simulink model "gm_gm_Encoder_test_interface"  (R2021b)
settings: Solver=FixedStepAuto  StartTime=0.0  StopTime=inf  RelTol=1e-3  EnableMultiTasking=on
undefined symbols (not defined in the file or in its folder): AXI4, Lite
libraries: axiinterfacelib x5, simulink x2
settings Model: Creator=Stijn  LastModifiedBy=Jeedella
settings SolverCC: ConcurrentTasks=on  AlgebraicLoopSolver=TrustRegion  PositivePriorityOrder=on
settings DataIOCC: ReturnWorkspaceOutputs=off
settings OptimizationCC: BlockReduction=off  ConditionallyExecuteInputs=off  EnhancedBackFolding=on  PassReuseOutputArgsAs=Individual arguments  MaxStackSize=64  OptimizeBlockOrder=speed  DifferentSizesBufferReuse=on  OptimizationCustomize=off  EfficientTunableParamExpr=on
settings DebuggingCC: AlgebraicLoopMsg=error  InheritedTsInSrcMsg=none  ParameterTunabilityLossMsg=error  SFMachineParentedDataDiag=warning  ArithmeticOperatorsInVariantConditions=warning
settings HardwareCC: ProdBitPerPointer=32  ProdBitPerSizeT=32  ProdBitPerPtrDiffT=32  ProdLargestAtomicInteger=Long  ProdLargestAtomicFloat=Double  ProdWordSize=32  ProdLongLongMode=on  ProdHWDeviceType=ARM Compatible->ARM Cortex  TargetBitPerPointer=64  TargetBitPerSizeT=64  TargetBitPerPtrDiffT=64  TargetLongLongMode=on  TargetIntDivRoundTo=Zero  TargetEndianess=LittleEndian  TargetWordSize=64  TargetHWDeviceType=Custom Processor->MATLAB Host Computer
settings ModelReferenceCC: ModelReferenceNumInstancesAllowed=Single
settings SFSimCC: MATLABDynamicMemAlloc=off  CustomCodeUndefinedFunction=UseInterfaceOnly
settings RTWCC: Description=Embedded Coder  SystemTargetFile=ert.tlc  HardwareBoard=Xilinx Zynq-7000 based board  TLCOptions="-aInlineSetEventsForThisBaseRateFcn=TLC_FALSE -aSuppressMultiTaskScheduler=TLC_FALSE  -aRateBasedStepFcn=0"  TemplateMakefile=ert_default_tmf  GenerateReport=on  Toolchain=Linaro AArch32 Linux v6.3.1  IncludeHyperlinkInReport=on  LaunchReport=on  GenerateTraceInfo=on  GenerateTraceReport=on  GenerateTraceReportSl=on  GenerateTraceReportSf=on  GenerateTraceReportEml=on
settings CodeAppCC: ForceParamTrailComments=on  IgnoreCustomStorageClasses=off  OperatorAnnotations=on  SimulinkDataObjDesc=on  SFDataObjDesc=on  InsertBlockDesc=on

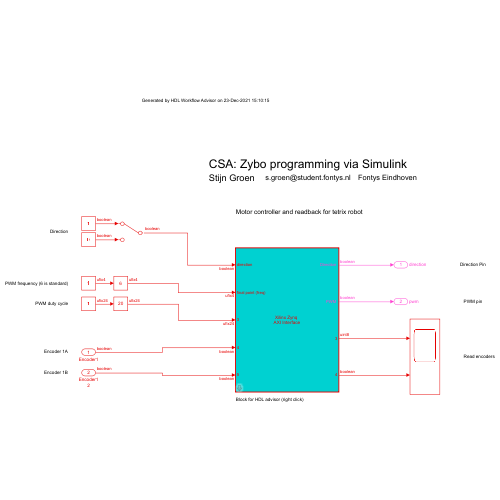
[thumbnail: Simulink's stored preview of the top-level diagram]
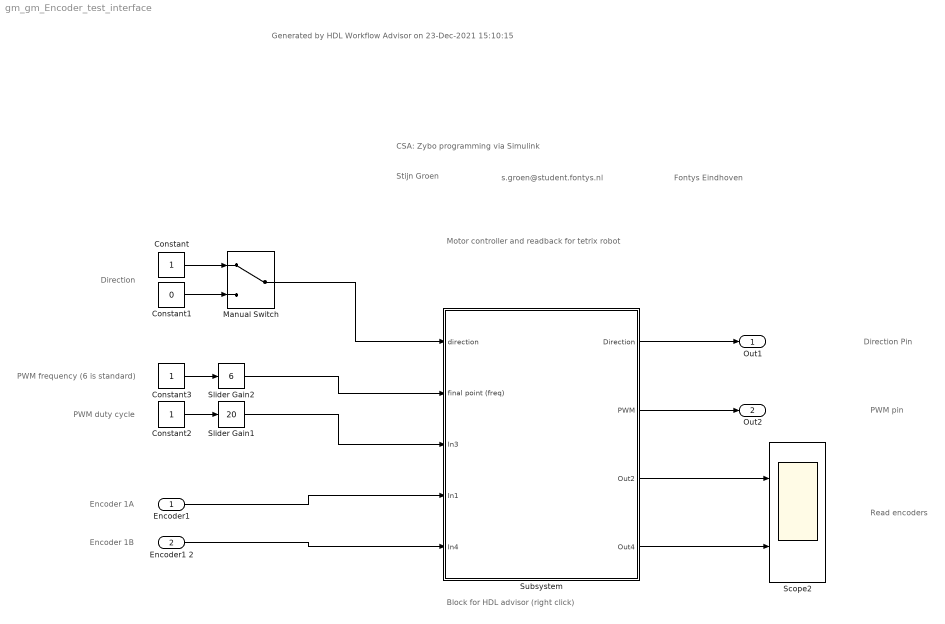
== system gm_gm_Encoder_test_interface ==
  note: Motor controller and readback for tetrix robot
  note: Read encoders
  note: PWM pin
  note: Direction Pin
  note: Encoder 1B
  note: Encoder 1A
  note: PWM duty cycle
  note: PWM frequency (6 is standard)
  note: Direction
  note: Block for HDL advisor (right click)
  note: Fontys Eindhoven
  note: s.groen@student.fontys.nl
  note: Stijn Groen
  note: CSA: Zybo programming via Simulink
  note: Generated by HDL Workflow Advisor on 23-Dec-2021 15:10:15
  "Encoder1 " : Inport  OutDataTypeStr=boolean
  Encoder1 2 : Inport  Port=2  OutDataTypeStr=boolean
  Constant : Constant  OutDataTypeStr=boolean  SampleTime=-1
  Constant1 : Constant  Value=0  OutDataTypeStr=boolean  SampleTime=-1
  Constant2 : Constant  OutDataTypeStr=fixdt(0,24,0)  SampleTime=-1
  Constant3 : Constant  OutDataTypeStr=fixdt(0,4,0)  SampleTime=-1
  Manual Switch : ManualSwitch
  Scope2 : Scope  NumInputPorts=2
  Slider Gain1 : simulink/Math Operations/Slider Gain  gain=20  low=0  high=100
  Slider Gain2 : simulink/Math Operations/Slider Gain  gain=6  low=0  high=15
  Subsystem : Subsystem  TreatAsAtomicUnit=on  mask(AXI4-Lite/AXI4 Interface){}
      mask help:
      | This is an automatically generated subsystem block.
      | This contains the AXI interface blocks that communicate with the Subsystem_ip IPCore generated from gm_Encoder_test/Subsystem subsystem.
      mask Display: disp(sprintf('Xilinx Zynq \nAXI Interface'));
  Out1 : Outport  SignalName=direction  VectorParamsAs1DForOutWhenUnconnected=off
  Out2 : Outport  Port=2  SignalName=pwm  VectorParamsAs1DForOutWhenUnconnected=off
  wires:
  Constant/1 -> Manual Switch/1
  Constant1/1 -> Manual Switch/2
  Constant3/1 -> Slider Gain2/1
  Manual Switch/1 -> Subsystem/1("direction ")
  Subsystem/1("Direction ") -> Out1/1
  Subsystem/2("PWM ") -> Out2/1
  Slider Gain2/1 -> Subsystem/2("final point (freq) ")
  Slider Gain1/1 -> Subsystem/3(In3)
  Constant2/1 -> Slider Gain1/1
  Subsystem/3(Out2) -> Scope2/1
  "Encoder1 "/1 -> Subsystem/4(In1)
  Encoder1 2/1 -> Subsystem/5(In4)
  Subsystem/4(Out4) -> Scope2/2

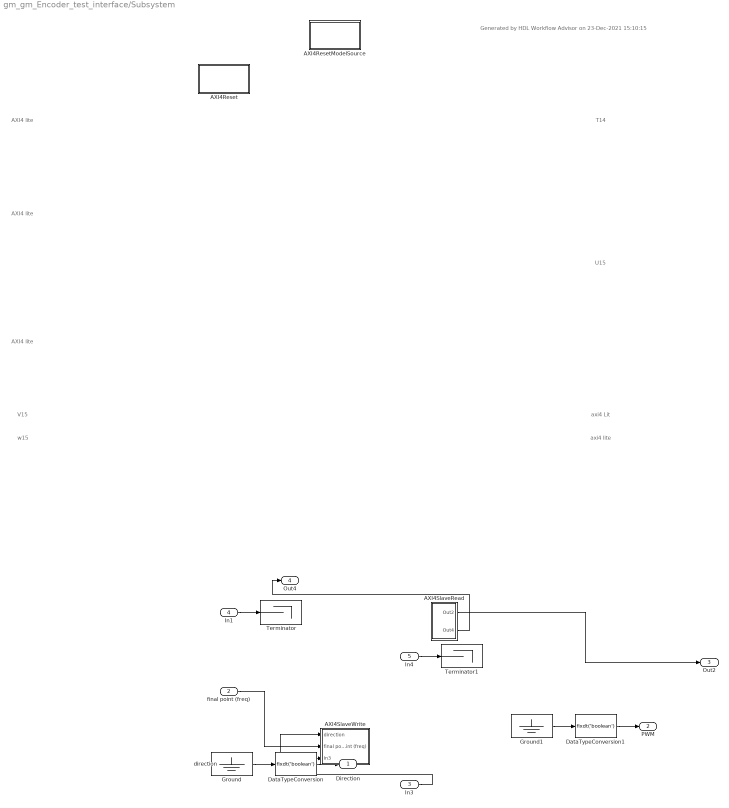
== system gm_gm_Encoder_test_interface/Subsystem ==
  note: T14
  note: U15
  note: axi4 Lit
  note: axi4 lite
  note: w15
  note: V15
  note: AXI4 lite
  note: AXI4 lite
  note: AXI4 lite
  note: Generated by HDL Workflow Advisor on 23-Dec-2021 15:10:15
  "direction " : Inport  OutDataTypeStr=boolean  PortDimensions=1  SampleTime=0.0002
  "final point (freq) " : Inport  Port=2  OutDataTypeStr=fixdt(0, 4, 0)  PortDimensions=1  SampleTime=0.0002
  In3 : Inport  Port=3  OutDataTypeStr=fixdt(0, 24, 0)  PortDimensions=1  SampleTime=0.0002
  In1 : Inport  Port=4  OutDataTypeStr=boolean  PortDimensions=1  SampleTime=0.0002
  In4 : Inport  Port=5  OutDataTypeStr=boolean  PortDimensions=1  SampleTime=0.0002
  AXI4Reset : Subsystem  mask(System Start){ShowInLibBrowser=0}
      mask prompts: ShowInLibBrowser "Simulink:masks:CustCodeMaskParam1_MP"
      settings: CopyFcn=cccopyfcn(gcb)  OpenFcn=ccopenfcn('System Start Function')
      mask Help: eval('feval(''rtwprivate'',''rtwhelpview'',''rtw_sys_start_block'')');
      mask Display: disp('System\nStart');
  AXI4ResetModelSource : Subsystem  mask(Model Source){ShowInLibBrowser=0}
      mask prompts: ShowInLibBrowser "Simulink:masks:CustCodeMaskParam1_MP"
      settings: CopyFcn=cccopyfcn(gcb)  OpenFcn=ccopenfcn('Model Source')
      mask Help: eval('feval(''rtwprivate'',''rtwhelpview'',''rtw_model_source_block'')');
      mask Display: disp('Model\nSource');
  AXI4SlaveRead : Subsystem  Priority=10
  AXI4SlaveWrite : Subsystem  Priority=1
  DataTypeConversion : DataTypeConversion  OutDataTypeStr=fixdt('boolean')  ConvertRealWorld=Stored Integer (SI)
  DataTypeConversion1 : DataTypeConversion  OutDataTypeStr=fixdt('boolean')  ConvertRealWorld=Stored Integer (SI)
  Ground : Ground
  Ground1 : Ground
  Terminator : Terminator
  Terminator1 : Terminator
  "Direction " : Outport  VectorParamsAs1DForOutWhenUnconnected=off
  "PWM " : Outport  Port=2  VectorParamsAs1DForOutWhenUnconnected=off
  Out2 : Outport  Port=3  VectorParamsAs1DForOutWhenUnconnected=off
  Out4 : Outport  Port=4  VectorParamsAs1DForOutWhenUnconnected=off
  wires:
  "direction "/1 -> AXI4SlaveWrite/1("direction ")
  "final point (freq) "/1 -> AXI4SlaveWrite/2("final point (freq) ")
  In3/1 -> AXI4SlaveWrite/3(In3)
  AXI4SlaveRead/1(Out2) -> Out2/1
  AXI4SlaveRead/2(Out4) -> Out4/1
  In1/1 -> Terminator/1
  In4/1 -> Terminator1/1
  DataTypeConversion/1 -> "Direction "/1
  Ground/1 -> DataTypeConversion/1
  DataTypeConversion1/1 -> "PWM "/1
  Ground1/1 -> DataTypeConversion1/1

== system gm_gm_Encoder_test_interface/Subsystem/AXI4Reset ==

== system gm_gm_Encoder_test_interface/Subsystem/AXI4ResetModelSource ==

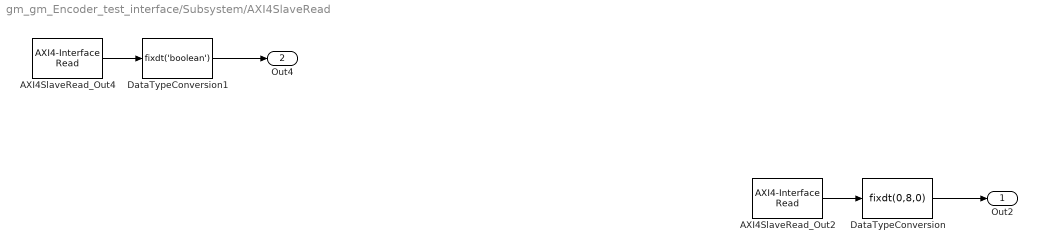
== system gm_gm_Encoder_test_interface/Subsystem/AXI4SlaveRead ==
  AXI4SlaveRead_Out2 : axiinterfacelib/AXI4-Interface Read  Priority=3  AXIInterfaceType=AXI4-Lite  DeviceName=/dev/mwipcore  RegisterOffset=hex2dec('10C')  DataLength=1  DataType=uint32  SampleTime=-1  blockPlatform=ZYNQ  SimulateUsing=Interpreted Execution
      settings: SourceProductBaseCode=ECZYNQ7000
  AXI4SlaveRead_Out4 : axiinterfacelib/AXI4-Interface Read  Priority=4  AXIInterfaceType=AXI4-Lite  DeviceName=/dev/mwipcore  RegisterOffset=hex2dec('110')  DataLength=1  DataType=uint32  SampleTime=-1  blockPlatform=ZYNQ  SimulateUsing=Interpreted Execution
      settings: SourceProductBaseCode=ECZYNQ7000
  DataTypeConversion : DataTypeConversion  OutDataTypeStr=fixdt(0,8,0)  ConvertRealWorld=Stored Integer (SI)
  DataTypeConversion1 : DataTypeConversion  OutDataTypeStr=fixdt('boolean')  ConvertRealWorld=Stored Integer (SI)
  Out2 : Outport  VectorParamsAs1DForOutWhenUnconnected=off
  Out4 : Outport  Port=2  VectorParamsAs1DForOutWhenUnconnected=off
  wires:
  AXI4SlaveRead_Out2/1 -> DataTypeConversion/1
  DataTypeConversion1/1 -> Out4/1
  DataTypeConversion/1 -> Out2/1
  AXI4SlaveRead_Out4/1 -> DataTypeConversion1/1

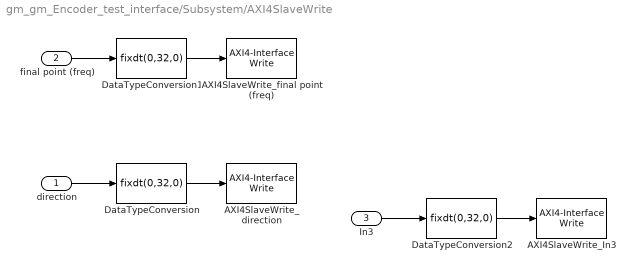
== system gm_gm_Encoder_test_interface/Subsystem/AXI4SlaveWrite ==
  "direction " : Inport  OutDataTypeStr=boolean  PortDimensions=1  SampleTime=0.0002
  "final point (freq) " : Inport  Port=2  OutDataTypeStr=fixdt(0, 4, 0)  PortDimensions=1  SampleTime=0.0002
  In3 : Inport  Port=3  OutDataTypeStr=fixdt(0, 24, 0)  PortDimensions=1  SampleTime=0.0002
  AXI4SlaveWrite_In3 : axiinterfacelib/AXI4-Interface Write  Priority=4  AXIInterfaceType=AXI4-Lite  DeviceName=/dev/mwipcore  RegisterOffset=hex2dec('108')  blockPlatform=ZYNQ  SimulateUsing=Interpreted execution
      settings: SourceProductBaseCode=ECZYNQ7000
  "AXI4SlaveWrite_direction " : axiinterfacelib/AXI4-Interface Write  Priority=2  AXIInterfaceType=AXI4-Lite  DeviceName=/dev/mwipcore  RegisterOffset=hex2dec('100')  blockPlatform=ZYNQ  SimulateUsing=Interpreted execution
      settings: SourceProductBaseCode=ECZYNQ7000
  "AXI4SlaveWrite_final point (freq) " : axiinterfacelib/AXI4-Interface Write  Priority=3  AXIInterfaceType=AXI4-Lite  DeviceName=/dev/mwipcore  RegisterOffset=hex2dec('104')  blockPlatform=ZYNQ  SimulateUsing=Interpreted execution
      settings: SourceProductBaseCode=ECZYNQ7000
  DataTypeConversion : DataTypeConversion  OutDataTypeStr=fixdt(0,32,0)  ConvertRealWorld=Stored Integer (SI)
  DataTypeConversion1 : DataTypeConversion  OutDataTypeStr=fixdt(0,32,0)  ConvertRealWorld=Stored Integer (SI)
  DataTypeConversion2 : DataTypeConversion  OutDataTypeStr=fixdt(0,32,0)  ConvertRealWorld=Stored Integer (SI)
  wires:
  "final point (freq) "/1 -> DataTypeConversion1/1
  In3/1 -> DataTypeConversion2/1
  "direction "/1 -> DataTypeConversion/1
  DataTypeConversion2/1 -> AXI4SlaveWrite_In3/1
  DataTypeConversion/1 -> "AXI4SlaveWrite_direction "/1
  DataTypeConversion1/1 -> "AXI4SlaveWrite_final point (freq) "/1
